simulink model "System_TargetTracking_EKF_Simulation"  (Simulink 6.3)
settings: Solver=VariableStepDiscrete  StartTime=0.0  StopTime=50.0  RelTol=1e-3
libraries: simulink x2
settings Model: LastModifiedBy=Huang

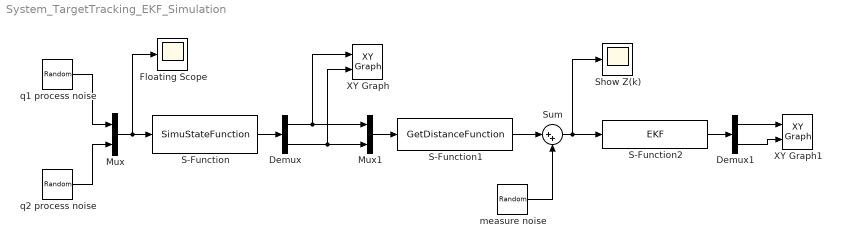
== system System_TargetTracking_EKF_Simulation ==
  Demux : Demux  Outputs=2
  Demux1 : Demux  Outputs=2
  Floating Scope : Scope
      settings: TimeRange=10  YMin=-3  YMax=2
  Mux : Mux  Description=Mux  Inputs=2
  Mux1 : Mux  Inputs=2
  S-Function : S-Function  FunctionName=SimuStateFunction
  S-Function1 : S-Function  FunctionName=GetDistanceFunction
  S-Function2 : S-Function  FunctionName=EKF
  Show Z(k) : Scope
      settings: SaveName=ScopeData3
  Sum : Sum  Inputs=|++
  XY Graph : simulink/Sinks/XY Graph  xmin=0  xmax=50  ymin=-5  ymax=25  st=1
  XY Graph1 : simulink/Sinks/XY Graph  xmin=0  xmax=50  ymin=-5  ymax=25  st=1
  measure noise : RandomNumber  SampleTime=1
  q1 process noise : RandomNumber  Variance=0.01  Seed=3  SampleTime=1
  q2 process noise : RandomNumber  Variance=0.04  Seed=10  SampleTime=1
  wires:
  q1 process noise/1 -> Mux/1
  q2 process noise/1 -> Mux/2
  Mux/1 -> Floating Scope/1, S-Function/1
  S-Function/1 -> Demux/1
  Demux/1 -> Mux1/1, XY Graph/1
  Mux1/1 -> S-Function1/1
  S-Function1/1 -> Sum/1
  measure noise/1 -> Sum/2
  Sum/1 -> Show Z(k)/1, S-Function2/1
  Demux/2 -> Mux1/2, XY Graph/2
  Demux1/1 -> XY Graph1/1
  Demux1/2 -> XY Graph1/2
  S-Function2/1 -> Demux1/1
